simulink library "medusa5h1"  (R2022b)
settings: Solver=VariableStepAuto  StartTime=0.0  StopTime=10.0  RelTol=1e-3
values from neighbouring files (symbols this model uses):
  MedusaConfig = struct('BandSplitConfig', BandSplitConfig,                            'DRFDPConfig', DRFDPConfig,                            'FRFDPConfig', FRFDPConfig,                            'SurroundConfig', SurroundConfig,                            'MSConfig', MSConfig,                            'PremixConfig', PremixConfig.Stereo,                            'PremixTune', PremixTune.Stereo,               ...(+1303 chars)    [medusa5h1_init.m]
undefined symbols (not defined in the file or in its folder): Row
libraries: MedusaDelays x14, TuneVar x11, FeaturePath x4, TOP x3, BassManager x1, MedusaCaeEnable x1, TrebleBoost x1, MedusaBandSplit x1, MedusaFDP x1, MedusaFullRateFDP x1, MonoDetector x1, MedusaSPUMDecayEst x1
settings Model: Creator=ud1041536  LastModifiedBy=jk1043656
settings SolverCC: AlgebraicLoopSolver=TrustRegion
settings DebuggingCC: UnconnectedInputMsg=warning  UnconnectedOutputMsg=warning  UnconnectedLineMsg=warning  SFMachineParentedDataDiag=warning  ArithmeticOperatorsInVariantConditions=warning
settings ModelReferenceCC: EnableRefExpFcnMdlSchedulingChecks=on
settings SFSimCC: CustomCodeUndefinedFunction=UseInterfaceOnly

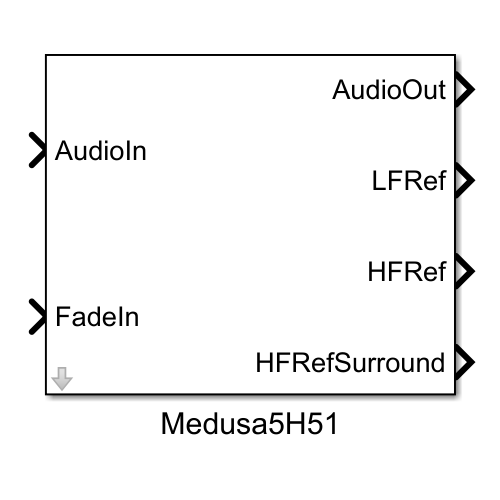
[thumbnail: Simulink's stored preview of the top-level diagram]
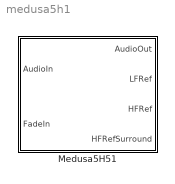
== system medusa5h1 ==
  Medusa5H51 : Subsystem  mask{config=MedusaConfig}
      mask prompts: config "Config struct name:"
      mask init:
      | tailCompEQ = config.tailCompEQ;
      | % delayConfig = config.DelayConfig;
      | 
      | % % Set 2 Medusa parts to be atomic if in Indirect Addressing Mode
      | % isIndirect = CoreIndexMask.IsIndirectAddressing(gcbh);
      | % if isIndirect
      | %     atomicSetting = 'on';
      | % else
      | %     atomicSetting = 'off';
      | % end
      | % p1Name = MaskUtil.SubBlockName(gcbh, 'Medusa5H1 Part 1');
      | % p2Name = MaskUtil.SubBlockName(gcbh, 'Medusa5H1 Part 2');
      | % 
      | % if -1 ~= (getSimulinkBlockHandle(p1Name))
      | %     MaskUtil.safe_setparam(p1Name, 'TreatAsAtomicUnit', atomicSetting);
      | % end
      | % 
      | % if -1 ~= (getSimulinkBlockHandle(p2Name))
      | %     MaskUtil.safe_setparam(p2Name, 'TreatAsAtomicUnit', atomicSetting);
      | % end

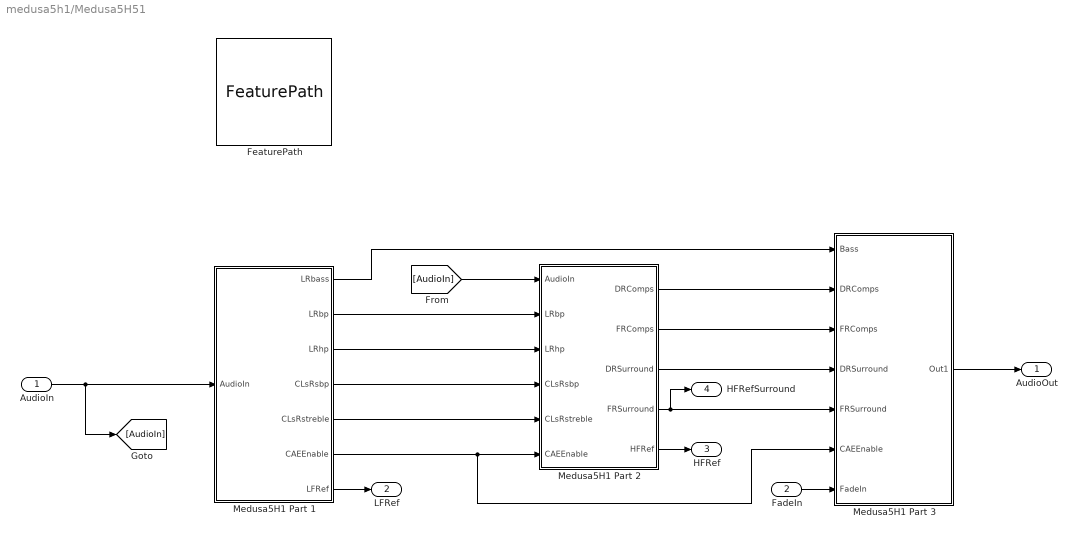
== system medusa5h1/Medusa5H51 ==
  AudioIn : Inport
  FadeIn : Inport  Port=2  OutDataTypeStr=single
  FeaturePath : FeaturePath/FeaturePath  FeatureName=Medusa  IsGroup=off  GroupNumber=-1  IsModule=off  TriggerInit=[620 344 735 451]
      settings: SourceProductName=Bose Talaria
  Medusa5H1 Part 1 : Subsystem  TreatAsAtomicUnit=on
      settings: RTWSystemCode=Nonreusable function
  Medusa5H1 Part 2 : Subsystem  TreatAsAtomicUnit=on
      settings: RTWSystemCode=Nonreusable function
  Medusa5H1 Part 3 : Subsystem  TreatAsAtomicUnit=on
      settings: RTWSystemCode=Nonreusable function  FunctionWithSeparateData=on
  AudioOut : Outport  VectorParamsAs1DForOutWhenUnconnected=off
  LFRef : Outport  Port=2
  HFRef : Outport  Port=3
  HFRefSurround : Outport  Port=4
  wires:
  Medusa5H1 Part 2/5(HFRef) -> HFRef/1
  Medusa5H1 Part 1/7(LFRef) -> LFRef/1
  Medusa5H1 Part 1/4(CLsRsbp) -> Medusa5H1 Part 2/4(CLsRsbp)
  Medusa5H1 Part 2/3(DRSurround) -> Medusa5H1 Part 3/4(DRSurround)
  Medusa5H1 Part 2/4(FRSurround) -> HFRefSurround/1, Medusa5H1 Part 3/5(FRSurround)
  Medusa5H1 Part 1/5(CLsRstreble) -> Medusa5H1 Part 2/5(CLsRstreble)
  Medusa5H1 Part 1/1(LRbass) -> Medusa5H1 Part 3/1(Bass)
  Medusa5H1 Part 2/1(DRComps) -> Medusa5H1 Part 3/2(DRComps)
  Medusa5H1 Part 2/2(FRComps) -> Medusa5H1 Part 3/3(FRComps)
  FadeIn/1 -> Medusa5H1 Part 3/7(FadeIn)
  Medusa5H1 Part 3/1(Out1) -> AudioOut/1
  Medusa5H1 Part 1/2(LRbp) -> Medusa5H1 Part 2/2(LRbp)
  Medusa5H1 Part 1/3(LRhp) -> Medusa5H1 Part 2/3(LRhp)
  AudioIn/1 -> Medusa5H1 Part 1/1(AudioIn), [AudioIn]
  [AudioIn] -> Medusa5H1 Part 2/1(AudioIn)
  Medusa5H1 Part 1/6(CAEEnable) -> Medusa5H1 Part 3/6(CAEEnable), Medusa5H1 Part 2/6(CAEEnable)

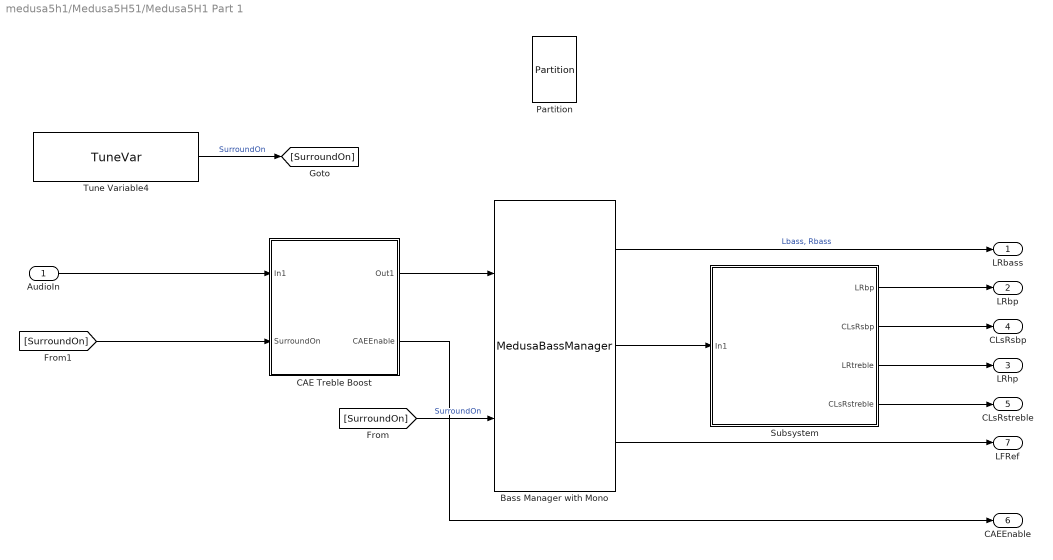
== system medusa5h1/Medusa5H51/Medusa5H1 Part 1 ==
  AudioIn : Inport
  Bass Manager with Mono : BassManager/MedusaBassManager  Config=Config.BassManager
  CAE Treble Boost : Subsystem  Variant=on
  Partition : FeaturePath/Partition  PartitionNumber=2  TriggerInit=[505 -119 550 -51]
      settings: SourceProductName=Bose Talaria
  Subsystem : Subsystem  TreatAsAtomicUnit=on  RTWFileName=MedusaBandSplit
      settings: RTWSystemCode=Nonreusable function  RTWFileNameOpts=User specified  FunctionWithSeparateData=on
  Tune Variable4 : TuneVar/TuneVar  Description=|  TuneName=SurroundOn  SpecifyMaxSize=off  VariableDim=1 (Row)  MaxSize=[1 1]  TunabilityNumber=1  MinValue=[]  MaxValue=[]  TriggerInit=[-10 -10 160 40]  MaskValue=2
      | General surround control parameter
      | STEREO_MODE = 0
      | SURROUND_PASSTHRU_MODE = 1
      | MEDUSA_2_CHANNEL_MODE = 2
      | MEDUSA_5_1_MODE = 3
      settings: SourceProductName=Bose Talaria
  LRbass : Outport  VectorParamsAs1DForOutWhenUnconnected=off
  LRbp : Outport  Port=2  VectorParamsAs1DForOutWhenUnconnected=off
  LRhp : Outport  Port=3  VectorParamsAs1DForOutWhenUnconnected=off
  CLsRsbp : Outport  Port=4  VectorParamsAs1DForOutWhenUnconnected=off
  CLsRstreble : Outport  Port=5  VectorParamsAs1DForOutWhenUnconnected=off
  CAEEnable : Outport  Port=6
  LFRef : Outport  Port=7
  wires:
  Bass Manager with Mono/3 -> LFRef/1
  Subsystem/2(CLsRsbp) -> CLsRsbp/1
  Subsystem/3(LRtreble) -> LRhp/1
  Subsystem/4(CLsRstreble) -> CLsRstreble/1
  [SurroundOn] -> Bass Manager with Mono/2  "SurroundOn"
  Bass Manager with Mono/2 -> Subsystem/1(In1)
  Subsystem/1(LRbp) -> LRbp/1
  Bass Manager with Mono/1 -> LRbass/1  "Lbass, Rbass"
  AudioIn/1 -> CAE Treble Boost/1(In1)
  Tune Variable4/1 -> [SurroundOn]  "SurroundOn"
  [SurroundOn] -> CAE Treble Boost/2(SurroundOn)
  CAE Treble Boost/2(CAEEnable) -> CAEEnable/1
  CAE Treble Boost/1(Out1) -> Bass Manager with Mono/1

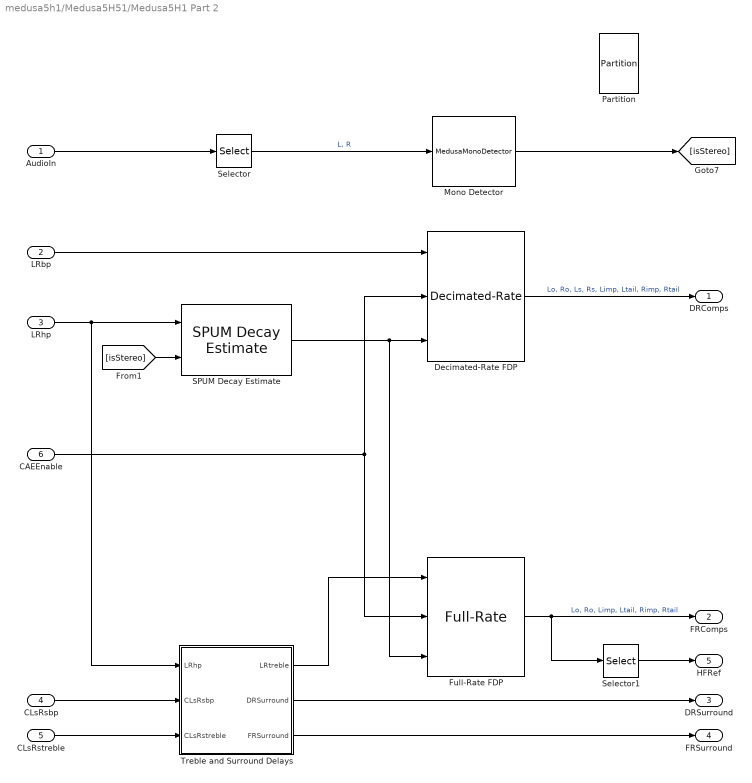
== system medusa5h1/Medusa5H51/Medusa5H1 Part 2 ==
  AudioIn : Inport  OutDataTypeStr=single
  LRbp : Inport  Port=2
  LRhp : Inport  Port=3
  CLsRsbp : Inport  Port=4
  CLsRstreble : Inport  Port=5
  CAEEnable : Inport  Port=6
  Decimated-Rate FDP : MedusaFDP/Decimated-Rate  FeatureName=DeciRate  configStruct=config.DRFDPConfig
  Full-Rate FDP : MedusaFullRateFDP/Full-Rate  FeatureName=FullRate  configStruct=config.FRFDPConfig
  Mono Detector : MonoDetector/MedusaMonoDetector  Config=Config.MonoDetector
  Partition : FeaturePath/Partition  PartitionNumber=3  TriggerInit=[1260 261 1305 329]
      settings: SourceProductName=Bose Talaria
  SPUM Decay Estimate : MedusaSPUMDecayEst/SPUM Decay Estimate  configStruct=config.FRFDPConfig
  Selector : Selector  NumberOfDimensions=2  InputPortWidth=3  IndexOptions=Select all,Index vector (dialog)  Indices=[1 3],[1,2]  OutputSizes=1,1
  Selector1 : Selector  NumberOfDimensions=2  InputPortWidth=3  IndexOptions=Select all,Index vector (dialog)  Indices=[1 3],[1 2 3 5]  OutputSizes=1,1
  Treble and Surround Delays : Subsystem  TreatAsAtomicUnit=on
      settings: RTWSystemCode=Nonreusable function  FunctionWithSeparateData=on
  DRComps : Outport  VectorParamsAs1DForOutWhenUnconnected=off
  FRComps : Outport  Port=2  VectorParamsAs1DForOutWhenUnconnected=off
  DRSurround : Outport  Port=3  VectorParamsAs1DForOutWhenUnconnected=off
  FRSurround : Outport  Port=4  VectorParamsAs1DForOutWhenUnconnected=off
  HFRef : Outport  Port=5
  wires:
  Selector1/1 -> HFRef/1
  Full-Rate FDP/1 -> FRComps/1, Selector1/1  "Lo, Ro, Limp, Ltail, Rimp, Rtail"
  Decimated-Rate FDP/1 -> DRComps/1  "Lo, Ro, Ls, Rs, Limp, Ltail, Rimp, Rtail"
  SPUM Decay Estimate/1 -> Full-Rate FDP/3, Decimated-Rate FDP/3
  CAEEnable/1 -> Decimated-Rate FDP/2, Full-Rate FDP/2
  Mono Detector/1 -> [isStereo]
  Selector/1 -> Mono Detector/1  "L, R"
  AudioIn/1 -> Selector/1
  LRbp/1 -> Decimated-Rate FDP/1
  LRhp/1 -> Treble and Surround Delays/1(LRhp), SPUM Decay Estimate/1
  [isStereo] -> SPUM Decay Estimate/2
  Treble and Surround Delays/3(FRSurround) -> FRSurround/1
  CLsRsbp/1 -> Treble and Surround Delays/2(CLsRsbp)
  CLsRstreble/1 -> Treble and Surround Delays/3(CLsRstreble)
  Treble and Surround Delays/1(LRtreble) -> Full-Rate FDP/1
  Treble and Surround Delays/2(DRSurround) -> DRSurround/1

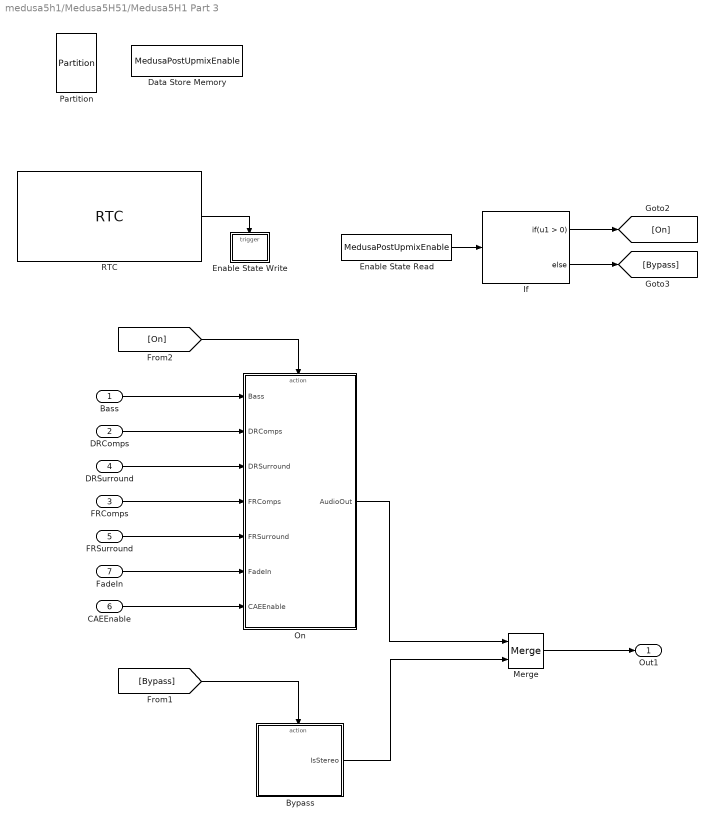
== system medusa5h1/Medusa5H51/Medusa5H1 Part 3 ==
  Bass : Inport
  DRComps : Inport  Port=2
  FRComps : Inport  Port=3
  DRSurround : Inport  Port=4
  FRSurround : Inport  Port=5
  CAEEnable : Inport  Port=6
  FadeIn : Inport  Port=7
  Bypass : Subsystem
  Data Store Memory : DataStoreMemory  DataStoreName=MedusaPostUpmixEnable  ReadBeforeWriteMsg=warning  WriteAfterWriteMsg=warning  WriteAfterReadMsg=warning  InitialValue=1  ShowAdditionalParam=off  OutDataTypeStr=uint32
  Enable State Read : DataStoreRead  DataStoreName=MedusaPostUpmixEnable  IndexOptions=Index vector (dialog)  Indices=1  OutputSizes=1
  Enable State Write : Subsystem
  If : If
  Merge : Merge  InitialOutput=MedusaConfig.outputDefault
  On : Subsystem
  Partition : FeaturePath/Partition  PartitionNumber=5  TriggerInit=[335 281 380 349]
      settings: SourceProductName=Bose Talaria
  RTC : RTC/RTC  REQ_Priority=RTC_Mask.NormalPriority  RequestAtInit=off  EnableRequest=on  REQElemType1=int32  REQElemWidth1=1  REQElemInitial1=[]  REQElemType2=uint32  REQElemWidth2=1  REQElemInitial2=[]  REQElemType3=uint32  REQElemWidth3=1  REQElemInitial3=[]  REQElemType4=uint32  REQElemWidth4=1  REQElemInitial4=[]  REQElemType5=uint32  REQElemWidth5=1  REQElemInitial5=[]  REQElemType6=uint32  REQElemWidth6=1  REQElemInitial6=[]  REQElemType7=uint32  REQElemWidth7=1  REQElemInitial7=[]  REQElemType8=uint32  REQElemWidth8=1  REQElemInitial8=[]  REQElemType9=uint32  REQElemWidth9=1  REQElemInitial9=[]  REQElemType10=uint32  REQElemWidth10=1  REQElemInitial10=[]  EnableResponse=on  EnableRSP_StatusIn=off  RSPElemType1=uint32  RSPElemWidth1=1  RSPElemType2=uint32  RSPElemWidth2=1  RSPElemType3=uint32  RSPElemWidth3=1  RSPElemType4=uint32  RSPElemWidth4=1  RSPElemType5=uint32  RSPElemWidth5=1  RSPElemType6=uint32  RSPElemWidth6=1  RSPElemType7=uint32  RSPElemWidth7=1  RSPElemType8=uint32  RSPElemWidth8=1  RSPElemType9=uint32  RSPElemWidth9=1  RSPElemType10=uint32  RSPElemWidth10=1  EnableNotification=off  EnableNTF_PrepTrig=off  NTFElemType1=uint32  NTFElemWidth1=1  NTFElemType2=uint32  NTFElemWidth2=1  NTFElemType3=uint32  NTFElemWidth3=1  NTFElemType4=uint32  NTFElemWidth4=1  NTFElemType5=uint32  NTFElemWidth5=1  NTFElemType6=uint32  NTFElemWidth6=1  NTFElemType7=uint32  NTFElemWidth7=1  NTFElemType8=uint32  NTFElemWidth8=1  NTFElemType9=uint32  NTFElemWidth9=1  NTFElemType10=uint32  NTFElemWidth10=1  MaskMessageName=PostUpmixDisable
      settings: SourceProductName=Bose Talaria
  Out1 : Outport  VectorParamsAs1DForOutWhenUnconnected=off
  wires:
  DRSurround/1 -> On/3(DRSurround)
  FRSurround/1 -> On/5(FRSurround)
  FadeIn/1 -> On/6(FadeIn)
  FRComps/1 -> On/4(FRComps)
  Bass/1 -> On/1(Bass)
  DRComps/1 -> On/2(DRComps)
  [Bypass] -> Bypass/Action
  Bypass/1(IsStereo) -> Merge/2
  On/1(AudioOut) -> Merge/1
  Merge/1 -> Out1/1
  If/1 -> [On]
  If/2 -> [Bypass]
  Enable State Read/1 -> If/1
  [On] -> On/Action
  RTC/1 -> Enable State Write/Trigger
  CAEEnable/1 -> On/7(CAEEnable)

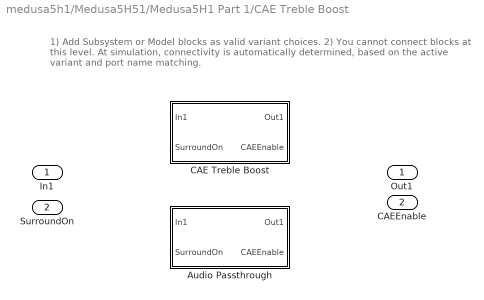
== system medusa5h1/Medusa5H51/Medusa5H1 Part 1/CAE Treble Boost ==
  note: 1) Add Subsystem or Model blocks as valid variant choices.
      | 2) You cannot connect blocks at this level. At simulation, connectivity is automatically
      | determined, based on the active variant and port name matching.
  In1 : Inport
  SurroundOn : Inport  Port=2
  Audio Passthrough : Subsystem  VariantControl=include_CAE == 0
  CAE Treble Boost : Subsystem  VariantControl=include_CAE == 1
  Out1 : Outport
  CAEEnable : Outport  Port=2

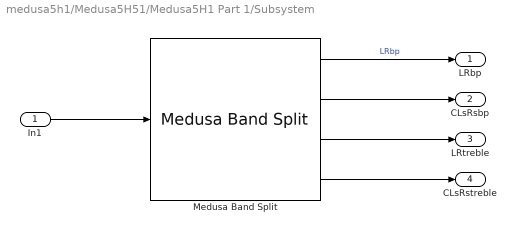
== system medusa5h1/Medusa5H51/Medusa5H1 Part 1/Subsystem ==
  In1 : Inport
  Medusa Band Split : MedusaBandSplit/Medusa Band Split  configStruct=config.BandSplitConfig
  LRbp : Outport  VectorParamsAs1DForOutWhenUnconnected=off
  CLsRsbp : Outport  Port=2  VectorParamsAs1DForOutWhenUnconnected=off
  LRtreble : Outport  Port=3  VectorParamsAs1DForOutWhenUnconnected=off
  CLsRstreble : Outport  Port=4  VectorParamsAs1DForOutWhenUnconnected=off
  wires:
  In1/1 -> Medusa Band Split/1
  Medusa Band Split/4 -> CLsRstreble/1
  Medusa Band Split/3 -> LRtreble/1
  Medusa Band Split/1 -> LRbp/1  "LRbp"
  Medusa Band Split/2 -> CLsRsbp/1

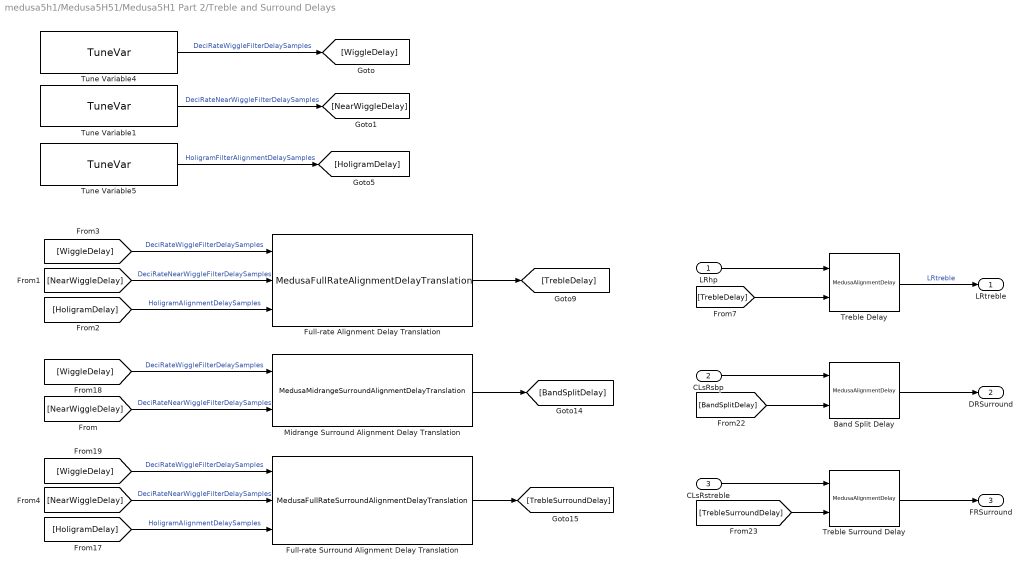
== system medusa5h1/Medusa5H51/Medusa5H1 Part 2/Treble and Surround Delays ==
  LRhp : Inport
  CLsRsbp : Inport  Port=2
  CLsRstreble : Inport  Port=3
  Band Split Delay : MedusaDelays/MedusaAlignmentDelay  Config=Config.Midrange51Delay
  Full-rate Alignment Delay Translation : MedusaDelays/MedusaFullRateAlignmentDelayTranslation  Config=Config.TrebleDelayTranslation
  Full-rate Surround Alignment Delay Translation : MedusaDelays/MedusaFullRateSurroundAlignmentDelayTranslation  Config=Config.Treble51DelayTranslation
  Midrange Surround Alignment Delay Translation : MedusaDelays/MedusaMidrangeSurroundAlignmentDelayTranslation  Config=Config.Midrange51DelayTranslation
  Treble Delay : MedusaDelays/MedusaAlignmentDelay  Config=Config.TrebleDelay
  Treble Surround Delay : MedusaDelays/MedusaAlignmentDelay  Config=Config.Treble51Delay
  Tune Variable1 : TuneVar/TuneVar  TuneName=DeciRateNearWiggleFilterDelaySamples  SpecifyMaxSize=off  VariableDim=1 (Row)  MaxSize=[1 1]  TunabilityNumber=1  MinValue=[]  MaxValue=[]  TriggerInit=[705 355 870 405]  MaskValue=Config.TrebleDelayTranslation.DefaultTuning.DeciRateNearWiggleDelay
      settings: SourceProductName=Bose Talaria
  Tune Variable4 : TuneVar/TuneVar  TuneName=DeciRateWiggleFilterDelaySamples  SpecifyMaxSize=off  VariableDim=1 (Row)  MaxSize=[1 1]  TunabilityNumber=1  MinValue=[]  MaxValue=[]  TriggerInit=[705 290 870 340]  MaskValue=Config.TrebleDelayTranslation.DefaultTuning.DeciRateWiggleDelay
      settings: SourceProductName=Bose Talaria
  Tune Variable5 : TuneVar/TuneVar  TuneName=HoligramFilterAlignmentDelaySamples  SpecifyMaxSize=off  VariableDim=1 (Row)  MaxSize=[1 1]  TunabilityNumber=1  MinValue=[]  MaxValue=[]  TriggerInit=[705 425 870 475]  MaskValue=Config.TrebleDelayTranslation.DefaultTuning.HoligramDelay
      settings: SourceProductName=Bose Talaria
  LRtreble : Outport
  DRSurround : Outport  Port=2
  FRSurround : Outport  Port=3
  wires:
  [WiggleDelay] -> Full-rate Surround Alignment Delay Translation/1  "DeciRateWiggleFilterDelaySamples"
  [TrebleDelay] -> Treble Delay/2
  Tune Variable1/1 -> [NearWiggleDelay]  "DeciRateNearWiggleFilterDelaySamples"
  [NearWiggleDelay] -> Full-rate Alignment Delay Translation/2  "DeciRateNearWiggleFilterDelaySamples"
  [HoligramDelay] -> Full-rate Surround Alignment Delay Translation/3  "HoligramAlignmentDelaySamples"
  [WiggleDelay] -> Full-rate Alignment Delay Translation/1  "DeciRateWiggleFilterDelaySamples"
  [NearWiggleDelay] -> Full-rate Surround Alignment Delay Translation/2  "DeciRateNearWiggleFilterDelaySamples"
  Tune Variable5/1 -> [HoligramDelay]  "HoligramFilterAlignmentDelaySamples"
  Treble Surround Delay/1 -> FRSurround/1
  [NearWiggleDelay] -> Midrange Surround Alignment Delay Translation/2  "DeciRateNearWiggleFilterDelaySamples"
  Tune Variable4/1 -> [WiggleDelay]  "DeciRateWiggleFilterDelaySamples"
  Full-rate Alignment Delay Translation/1 -> [TrebleDelay]
  [HoligramDelay] -> Full-rate Alignment Delay Translation/3  "HoligramAlignmentDelaySamples"
  [BandSplitDelay] -> Band Split Delay/2
  CLsRstreble/1 -> Treble Surround Delay/1
  LRhp/1 -> Treble Delay/1
  Full-rate Surround Alignment Delay Translation/1 -> [TrebleSurroundDelay]
  Band Split Delay/1 -> DRSurround/1
  CLsRsbp/1 -> Band Split Delay/1
  Midrange Surround Alignment Delay Translation/1 -> [BandSplitDelay]
  Treble Delay/1 -> LRtreble/1  "LRtreble"
  [WiggleDelay] -> Midrange Surround Alignment Delay Translation/1  "DeciRateWiggleFilterDelaySamples"
  [TrebleSurroundDelay] -> Treble Surround Delay/2

== system medusa5h1/Medusa5H51/Medusa5H1 Part 3/Bypass ==
  Action Port : ActionPort
  Constant : Constant  Value=MedusaConfig.outputDefault  OutDataTypeStr=single
  IsStereo : Outport  VectorParamsAs1DForOutWhenUnconnected=off
  wires:
  Constant/1 -> IsStereo/1

== system medusa5h1/Medusa5H51/Medusa5H1 Part 3/Enable State Write ==
  Trigger : TriggerPort  TriggerType=function-call  VariantControl=Variant  PortDimensions=1
  Constant : Constant  Value=0  OutDataTypeStr=uint32
  Data Store Write : DataStoreWrite  DataStoreName=MedusaPostUpmixEnable  IndexOptions=Index vector (dialog)  Indices=1  OutputSizes=1
  wires:
  Constant/1 -> Data Store Write/1

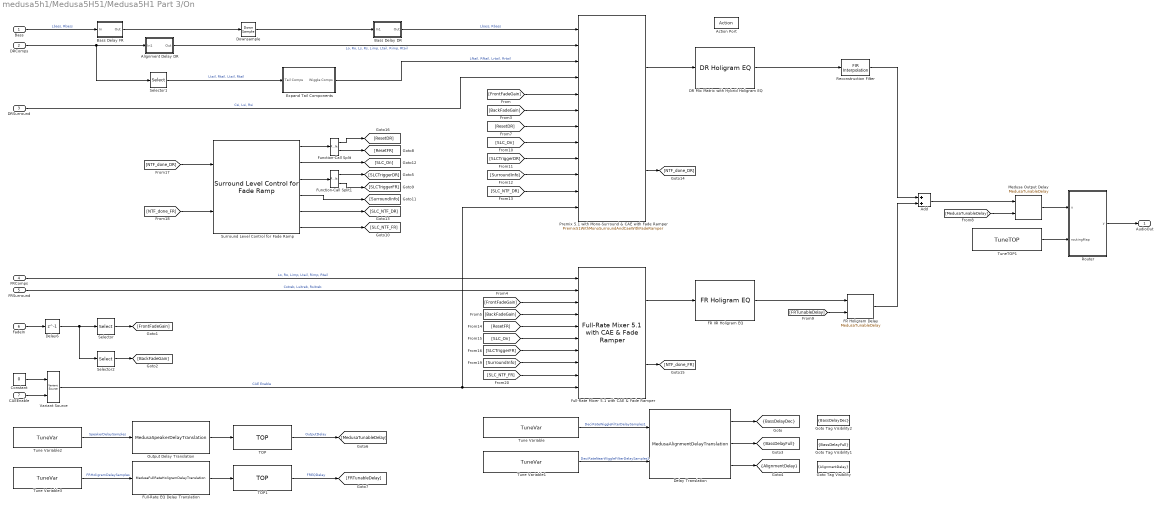
== system medusa5h1/Medusa5H51/Medusa5H1 Part 3/On ==
  Bass : Inport  OutDataTypeStr=single
  DRComps : Inport  Port=2  OutDataTypeStr=single
  DRSurround : Inport  Port=3
  FRComps : Inport  Port=4  OutDataTypeStr=single
  FRSurround : Inport  Port=5
  FadeIn : Inport  Port=6  OutDataTypeStr=single
  CAEEnable : Inport  Port=7
  Action Port : ActionPort
  Add : Sum
  Alignment Delay DR : Subsystem
      mask Display: disp 'Delay';
  Bass Delay DR : Subsystem
      mask Display: disp 'Delay DR';
  Bass Delay FR : Subsystem
      mask Display: disp 'Delay FR';
  Constant : Constant  Value=0  OutDataTypeStr=int32  SampleTime=-1
  DR Mix Matrix with Hybrid Holigram EQ : MedusaDRHoligramEQ/DR Holigram EQ  configStruct=config.HoligramEQConfig
  Delay Translation : MedusaDelays/MedusaAlignmentDelayTranslation  Config=Config.AlignmentDelayTranslation
  Delay6 : Delay  DelayLength=1  InitialCondition=1.0
  Downsample : DownSample  N=4
  Expand Tail Components : Subsystem  TreatAsAtomicUnit=on  RTWFileName=MedusaExpandTailComps
      settings: RTWSystemCode=Nonreusable function  RTWFileNameOpts=User specified  FunctionWithSeparateData=on
  FR Holigram Delay : MedusaDelays/MedusaTunableDelay  Config=Config.FullRateHoligramDelay
  FR IIR Holigram EQ : MedusaFRHoligramEQ/FR Holigram EQ  configStruct=config.HoligramEQConfig
  Full-Rate EQ Delay Translation : MedusaDelays/MedusaFullRateHoligramDelayTranslation  Config=Config.FullRateHoligramDelayTranslation
  Full-Rate Mixer 5.1 with CAE & Fade Ramper : MedusaFullRateMixer/Full-Rate Mixer 5.1 with CAE & Fade Ramper  MedusaFRMConfig=config.FRM5H1Config  MedusaFRMTune=config.FRM5H1Tune
  Function-Call Split : FunctionCallSplit  IconShape=distinctive  NumOutputPorts=2  OutputPortLayout=default
  Function-Call Split1 : FunctionCallSplit  IconShape=distinctive  NumOutputPorts=2  OutputPortLayout=default
  Goto Tag Visibility : GotoTagVisibility  GotoTag=AlignmentDelay
  Goto Tag Visibility1 : GotoTagVisibility  GotoTag=BassDelayFull
  Goto Tag Visibility2 : GotoTagVisibility  GotoTag=BassDelayDec
  Medusa Output Delay : MedusaDelays/MedusaTunableDelay  Config=Config.SpeakerDelay
  Output Delay Translation : MedusaDelays/MedusaSpeakerDelayTranslation  Config=Config.SpeakerDelayTranslation
  Premix 5.1 with Mono-Surround & CAE with Fade Ramper : MedusaPremix/Premix51WithMonoSurroundAndCaeWithFadeRamper  MedusaPremixConfig=config.Premix5H1Config  MedusaPremixTune=config.Premix5H1Tune  MSConfig=config.MSConfig
  Reconstruction Filter : dspmlti4/FIR Interpolation  FilterSource=Dialog parameters  PrivateCoeffs=0  h=config.BandSplitConfig.upfir  L=config.BandSplitConfig.D  FilterObject=FINTERP  InputProcessing=Columns as channels (frame based)  framing=Enforce single-rate processing  outputBufInitCond=0  roundingMode=Floor  overflowMode=off  firstCoeffDataTypeStr=Inherit: Same word length as input  firstCoeffMin=[]  firstCoeffMax=[]  firstCoeffLastDataTypeStr=Inherit: Same word length as input  outputDataTypeStr=Inherit: Same as accumulator  outputMin=[]  outputMax=[]  outputLastDataTypeStr=Inherit: Same as accumulator
  Router : MATLAB Function  TreatAsAtomicUnit=on
  Selector : Selector  NumberOfDimensions=2  InputPortWidth=2  IndexOptions=Index vector (dialog),Index vector (dialog)  Indices=1,1  OutputSizes=1,1
  Selector1 : Selector  NumberOfDimensions=2  InputPortWidth=3  IndexOptions=Select all,Index vector (dialog)  Indices=[1 3],[6 8 6 8]  OutputSizes=1,1
  Selector2 : Selector  NumberOfDimensions=2  InputPortWidth=2  IndexOptions=Index vector (dialog),Index vector (dialog)  Indices=1,2  OutputSizes=1,1
  Surround Level Control for Fade Ramp : MedusaSurroundLevelControl/Surround Level Control for Fade Ramp  SurroundConfig=config.SurroundConfig
  TOP : TOP/TOP  TriggerInit=[475 1205 620 1265]  TopName=OutputDelay  DataType=int32  BankNumber=0  PreOverlay=false  PostOverlay=false  Role=Automatic
      settings: SourceProductName=Bose Talaria
  TOP1 : TOP/TOP  TriggerInit=[475 1305 620 1365]  TopName=FREQDelay  DataType=int32  BankNumber=0  PreOverlay=false  PostOverlay=false  Role=Automatic
      settings: SourceProductName=Bose Talaria
  Tune Variable : TuneVar/TuneVar  TuneName=DeciRateWiggleFilterDelaySamples1  SpecifyMaxSize=off  VariableDim=1 (Row)  MaxSize=[1 1]  TunabilityNumber=1  MinValue=[]  MaxValue=[]  TriggerInit=[1095 1185 1330 1235]  MaskValue=Config.AlignmentDelayTranslation.DefaultTuning.DeciRateWiggleDelay
      settings: SourceProductName=Bose Talaria
  Tune Variable1 : TuneVar/TuneVar  TuneName=DeciRateNearWiggleFilterDelaySamples1  SpecifyMaxSize=off  VariableDim=1 (Row)  MaxSize=[1 1]  TunabilityNumber=1  MinValue=[]  MaxValue=[]  TriggerInit=[1095 1270 1330 1320]  MaskValue=Config.AlignmentDelayTranslation.DefaultTuning.DeciRateNearWiggleDelay
      settings: SourceProductName=Bose Talaria
  Tune Variable2 : TuneVar/TuneVar  TuneName=SpeakerDelaySamples  SpecifyMaxSize=off  VariableDim=1 (Row)  MaxSize=[]  TunabilityNumber=1  MinValue=[]  MaxValue=[]  TriggerInit=[-70 1210 100 1260]  MaskValue=Config.Get(@Config.SpeakerDelayTranslation.DefaultTuning.SpeakerDelay)
      settings: SourceProductName=Bose Talaria
  Tune Variable3 : TuneVar/TuneVar  TuneName=FRHoligramDelaySamples  SpecifyMaxSize=off  VariableDim=1 (Row)  MaxSize=[]  TunabilityNumber=1  MinValue=[]  MaxValue=[]  TriggerInit=[-70 1310 100 1360]  MaskValue=Config.Get(@Config.FullRateHoligramDelayTranslation.DefaultTuning.FullRateHoligramDelay)
      settings: SourceProductName=Bose Talaria
  TuneTOP1 : TuneVar/TuneTOP  TriggerInit=[2305 717 2475 773]  TopName=RoutingMap  TuneName=RoutingMap  DataType=single  TunabilityNumber=1  MinValue=[]  MaxValue=[]  BankNumber=0  PreOverlay=false  PostOverlay=false  UseSameName=on  MaskValue=config.routingMapDefault
      settings: SourceProductName=Bose Talaria
  Variant Source : VariantSource
  AudioOut : Outport  VectorParamsAs1DForOutWhenUnconnected=off
  tag scope: AlignmentDelay=scoped, BassDelayDec=scoped, BassDelayFull=scoped
  wires:
  Tune Variable/1 -> Delay Translation/1  "DeciRateWiggleFilterDelaySamples1"
  FRSurround/1 -> Full-Rate Mixer 5.1 with CAE & Fade Ramper/2  "Cstreb, Lsitreb, Rsitreb"
  DRSurround/1 -> Premix 5.1 with Mono-Surround & CAE with Fade Ramper/4  "Csi, Lsi, Rsi"
  Selector/1 -> [FrontFadeGain]
  Delay6/1 -> Selector/1, Selector2/1
  Selector2/1 -> [BackFadeGain]
  FadeIn/1 -> Delay6/1
  FR IIR Holigram EQ/1 -> FR Holigram Delay/1
  DR Mix Matrix with Hybrid Holigram EQ/1 -> Reconstruction Filter/1
  Medusa Output Delay/1 -> Router/1(u)
  FR Holigram Delay/1 -> Add/2
  Add/1 -> Medusa Output Delay/1
  TuneTOP1/1 -> Router/2(routingMap)
  Reconstruction Filter/1 -> Add/1
  Bass Delay FR/1(Out) -> Downsample/1
  Alignment Delay DR/1(Out) -> Premix 5.1 with Mono-Surround & CAE with Fade Ramper/2  "Lo, Ro, Ls, Rs, Limp, Ltail, Rimp, Rtail"
  DRComps/1 -> Alignment Delay DR/1(In1), Selector1/1
  Router/1(y) -> AudioOut/1
  Selector1/1 -> Expand Tail Components/1(Tail Comps)  "Ltail, Rtail, Ltail, Rtail"
  Bass/1 -> Bass Delay FR/1(In)  "Lbass, Rbass"
  Expand Tail Components/1(Wiggle Comps) -> Premix 5.1 with Mono-Surround & CAE with Fade Ramper/3  "Lftail, Rftail, Lrtail, Rrtail"
  [FrontFadeGain] -> Full-Rate Mixer 5.1 with CAE & Fade Ramper/3
  Premix 5.1 with Mono-Surround & CAE with Fade Ramper/1 -> DR Mix Matrix with Hybrid Holigram EQ/1
  [BackFadeGain] -> Full-Rate Mixer 5.1 with CAE & Fade Ramper/4
  Full-Rate Mixer 5.1 with CAE & Fade Ramper/1 -> FR IIR Holigram EQ/1
  Delay Translation/3 -> [AlignmentDelay]
  Delay Translation/2 -> [BassDelayFull]
  Delay Translation/1 -> [BassDelayDec]
  Tune Variable2/1 -> Output Delay Translation/1  "SpeakerDelaySamples"
  TOP/1 -> [MedusaTunableDelay]  "OutputDelay"
  Tune Variable3/1 -> Full-Rate EQ Delay Translation/1  "FRHoligramDelaySamples"
  [MedusaTunableDelay] -> Medusa Output Delay/2
  [FRTunableDelay] -> FR Holigram Delay/2
  Bass Delay DR/1(Out) -> Premix 5.1 with Mono-Surround & CAE with Fade Ramper/1  "Lbass, Rbass"
  Downsample/1 -> Bass Delay DR/1(In1)
  Output Delay Translation/1 -> TOP/1
  Full-Rate EQ Delay Translation/1 -> TOP1/1
  TOP1/1 -> [FRTunableDelay]  "FREQDelay"
  FRComps/1 -> Full-Rate Mixer 5.1 with CAE & Fade Ramper/1  "Lo, Ro, Limp, Ltail, Rimp, Rtail"
  [FrontFadeGain] -> Premix 5.1 with Mono-Surround & CAE with Fade Ramper/5
  [BackFadeGain] -> Premix 5.1 with Mono-Surround & CAE with Fade Ramper/6
  Surround Level Control for Fade Ramp/6 -> [SLC_NTF_FR]
  Surround Level Control for Fade Ramp/5 -> [SLC_NTF_DR]
  Function-Call Split/1 -> [ResetDR]
  Function-Call Split1/1 -> [SLCTriggerDR]
  Surround Level Control for Fade Ramp/4 -> [SurroundInfo]
  Function-Call Split/2 -> [ResetFR]
  Surround Level Control for Fade Ramp/2 -> [SLC_On]
  Function-Call Split1/2 -> [SLCTriggerFR]
  Surround Level Control for Fade Ramp/3 -> Function-Call Split1/1
  Surround Level Control for Fade Ramp/1 -> Function-Call Split/1
  [NTF_done_DR] -> Surround Level Control for Fade Ramp/1
  [NTF_done_FR] -> Surround Level Control for Fade Ramp/2
  [ResetDR] -> Premix 5.1 with Mono-Surround & CAE with Fade Ramper/7
  [SLC_On] -> Premix 5.1 with Mono-Surround & CAE with Fade Ramper/8
  [SLCTriggerDR] -> Premix 5.1 with Mono-Surround & CAE with Fade Ramper/9
  [SurroundInfo] -> Premix 5.1 with Mono-Surround & CAE with Fade Ramper/10
  [SLC_NTF_DR] -> Premix 5.1 with Mono-Surround & CAE with Fade Ramper/11
  [ResetFR] -> Full-Rate Mixer 5.1 with CAE & Fade Ramper/5
  [SLC_On] -> Full-Rate Mixer 5.1 with CAE & Fade Ramper/6
  [SLCTriggerFR] -> Full-Rate Mixer 5.1 with CAE & Fade Ramper/7
  [SurroundInfo] -> Full-Rate Mixer 5.1 with CAE & Fade Ramper/8
  [SLC_NTF_FR] -> Full-Rate Mixer 5.1 with CAE & Fade Ramper/9
  Premix 5.1 with Mono-Surround & CAE with Fade Ramper/2 -> [NTF_done_DR]
  Full-Rate Mixer 5.1 with CAE & Fade Ramper/2 -> [NTF_done_FR]
  CAEEnable/1 -> Variant Source/2
  Variant Source/1 -> Full-Rate Mixer 5.1 with CAE & Fade Ramper/10, Premix 5.1 with Mono-Surround & CAE with Fade Ramper/12  "CAE Enable"
  Constant/1 -> Variant Source/1
  Tune Variable1/1 -> Delay Translation/2  "DeciRateNearWiggleFilterDelaySamples1"

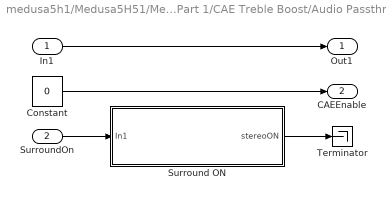
== system medusa5h1/Medusa5H51/Medusa5H1 Part 1/CAE Treble Boost/Audio Passthrough ==
  In1 : Inport
  SurroundOn : Inport  Port=2
  Constant : Constant  Value=0  OutDataTypeStr=int32  SampleTime=-1
  Surround ON : Subsystem
  Terminator : Terminator
  Out1 : Outport
  CAEEnable : Outport  Port=2
  wires:
  In1/1 -> Out1/1
  Constant/1 -> CAEEnable/1
  SurroundOn/1 -> Surround ON/1(In1)
  Surround ON/1(stereoON) -> Terminator/1

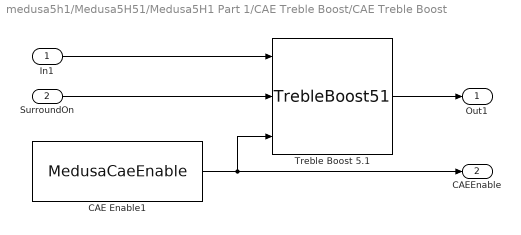
== system medusa5h1/Medusa5H51/Medusa5H1 Part 1/CAE Treble Boost/CAE Treble Boost ==
  In1 : Inport
  SurroundOn : Inport  Port=2
  CAE Enable1 : MedusaCaeEnable/MedusaCaeEnable  Config=[]  MaskMessageName=CAEEnable
  Treble Boost 5.1 : TrebleBoost/TrebleBoost51  Config=Config.TrebleBoost
  Out1 : Outport
  CAEEnable : Outport  Port=2
  wires:
  CAE Enable1/1 -> Treble Boost 5.1/3, CAEEnable/1
  Treble Boost 5.1/1 -> Out1/1
  SurroundOn/1 -> Treble Boost 5.1/2
  In1/1 -> Treble Boost 5.1/1

== system medusa5h1/Medusa5H51/Medusa5H1 Part 3/On/Alignment Delay DR ==
  In1 : Inport
  Alignment Delay DR : MedusaDelays/MedusaAlignmentDelay  Config=Config.MidrangeDelay
  Out : Outport
  wires:
  Alignment Delay DR/1 -> Out/1  "Lo, Ro, Ls, Rs, Limp, Ltail, Rimp, Rtail"
  In1/1 -> Alignment Delay DR/1
  [AlignmentDelay] -> Alignment Delay DR/2

== system medusa5h1/Medusa5H51/Medusa5H1 Part 3/On/Bass Delay DR ==
  In1 : Inport
  Bass Delay DR : MedusaDelays/MedusaAlignmentDelay  Config=Config.DeciRateBassDelay
  Out : Outport
  wires:
  Bass Delay DR/1 -> Out/1  "Lbass, Rbass"
  [BassDelayDec] -> Bass Delay DR/2
  In1/1 -> Bass Delay DR/1

== system medusa5h1/Medusa5H51/Medusa5H1 Part 3/On/Bass Delay FR ==
  In : Inport
  Bass Delay FR : MedusaDelays/MedusaAlignmentDelay  Config=Config.FullRateBassDelay
  Out : Outport
  wires:
  [BassDelayFull] -> Bass Delay FR/2
  Bass Delay FR/1 -> Out/1
  In/1 -> Bass Delay FR/1

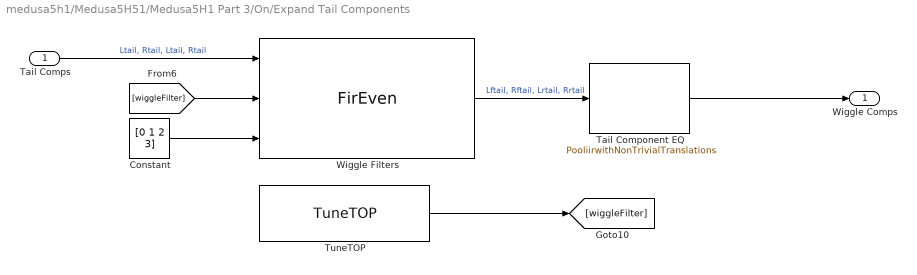
== system medusa5h1/Medusa5H51/Medusa5H1 Part 3/On/Expand Tail Components ==
  Tail Comps : Inport
  Constant : Constant  Value=[0 1 2 3]  OutDataTypeStr=single  SampleTime=-1
  Tail Component EQ : PooliirLib/PooliirwithNonTrivialTranslations  maxNumStages=tailCompEQ.maxNumStages  numStages=tailCompEQ.numStages  sosCoefficients=tailCompEQ.coeffs  variantType=tailCompEQ.variant  FeatureName=tailCompEQ
  TuneTOP : TuneVar/TuneTOP  TriggerInit=[265 167 435 223]  TopName=WiggleFilter  TuneName=WiggleFilter  DataType=single  TunabilityNumber=1  MinValue=[]  MaxValue=[]  BankNumber=0  PreOverlay=false  PostOverlay=false  UseSameName=on  MaskValue=config.wiggleFilterDefault
      settings: SourceProductName=Bose Talaria
  Wiggle Filters : FirEven/FirEven  Config=config.TailCompFirEvenSettings
      settings: SourceProductName=Bose Blocklib
  Wiggle Comps : Outport  VectorParamsAs1DForOutWhenUnconnected=off
  wires:
  [wiggleFilter] -> Wiggle Filters/2
  Wiggle Filters/1 -> Tail Component EQ/1  "Lftail, Rftail, Lrtail, Rrtail"
  TuneTOP/1 -> [wiggleFilter]
  Constant/1 -> Wiggle Filters/3
  Tail Component EQ/1 -> Wiggle Comps/1
  Tail Comps/1 -> Wiggle Filters/1  "Ltail, Rtail, Ltail, Rtail"

== system medusa5h1/Medusa5H51/Medusa5H1 Part 1/CAE Treble Boost/Audio Passthrough/Surround ON ==
  In1 : Inport
  TOP : TOP/TOP  TriggerInit=[440 20 585 80]  TopName=StereoON  DataType=int32  BankNumber=0  PreOverlay=false  PostOverlay=false  Role=Automatic
      settings: SourceProductName=Bose Talaria
  TranslateTrigger : TuneVar/TranslateTrigger  TriggerInit=[306 -100 344 -45]
      settings: SourceProductName=Bose Talaria
  Trivial Translation : MATLAB Function  TreatAsAtomicUnit=on
  stereoON : Outport  VectorParamsAs1DForOutWhenUnconnected=off
  wires:
  TOP/1 -> stereoON/1  "StereoON"
  In1/1 -> Trivial Translation/1(surroundOn)  "SurroundON"
  Trivial Translation/1(isStereo) -> TOP/1
  TranslateTrigger/1 -> Trivial Translation/Trigger

== matlab function medusa5h1/Medusa5H51/Medusa5H1 Part 3/On/Router ==
  data: u input; y output; routingMap input
function y = fcn(u, routingMap)

[frameSize, numIn] = size(u);
numOut = numel(routingMap);
y = coder.nullcopy(single(zeros(frameSize, numOut)));

for i = 1:numOut
    index = routingMap(i);
    if (index < 0) || (index >= numIn)
        y(:,i) = zeros(frameSize,1);
    else
        y(:,i) = u(:, index + 1); % add 1 for Matlab indexing
    end
end

== matlab function medusa5h1/Medusa5H51/Medusa5H1 Part 1/CAE Treble Boost/Audio Passthrough/Surround ON/Trivial Translation ==
  data: isStereo output; surroundOn input
  events: trigger input FUNCTION_CALL_EVENT
function isStereo  = checkStereo(surroundOn)
%#codegen

if(surroundOn.Value == 0 || surroundOn.Value == 2)
    isStereo = true;
else
    isStereo = false;
end
